simulink model "abe_simulink_model"  (R2022a)
settings: Solver=VariableStepAuto  StartTime=0.0  StopTime=50  RelTol=1e-3
libraries: simulink x1
settings Model: Creator=Abraham  LastModifiedBy=Abraham

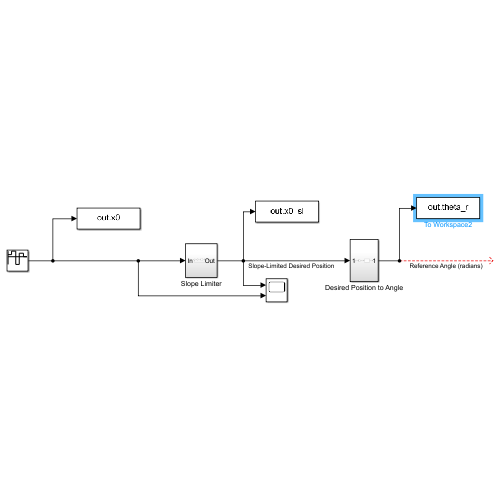
[thumbnail: Simulink's stored preview of the top-level diagram]
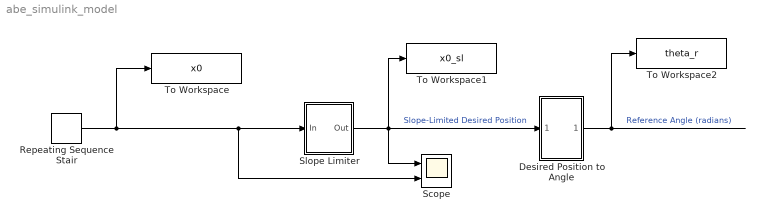
== system abe_simulink_model ==
  Desired Position to Angle : Subsystem
  Repeating Sequence Stair : simulink/Sources/Repeating Sequence Stair  OutValues=[5 15 -20 10 0].'  tsamp=10  OutMin=[]  OutMax=[]  OutDataTypeStr=double  OutputDataTypeScalingMode=double  OutDataType=fixdt(0,8)  ConRadixGroup=Best Precision: Vector-wise  OutScaling=2^-12
  Scope : Scope  NumInputPorts=2
  Slope Limiter : Subsystem
  To Workspace : ToWorkspace  VariableName=x0  SaveFormat=Timeseries  SampleTime=-1
  To Workspace1 : ToWorkspace  VariableName=x0_sl  SaveFormat=Timeseries  SampleTime=-1
  To Workspace2 : ToWorkspace  VariableName=theta_r  SaveFormat=Timeseries  SampleTime=-1
  wires:
  Slope Limiter/1(Out) -> To Workspace1/1, Desired Position to Angle/1(In1), Scope/1  "Slope-Limited Desired Position"
  Repeating Sequence Stair/1 -> To Workspace/1, Scope/2, Slope Limiter/1(In)
  Desired Position to Angle/1(Out1) -> To Workspace2/1  "Reference Angle (radians)"

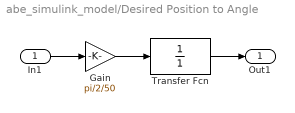
== system abe_simulink_model/Desired Position to Angle ==
  In1 : Inport
  Gain : Gain  Gain=pi/2/50
  Transfer Fcn : TransferFcn  Denominator=[1]
  Out1 : Outport
  wires:
  Gain/1 -> Transfer Fcn/1
  In1/1 -> Gain/1
  Transfer Fcn/1 -> Out1/1

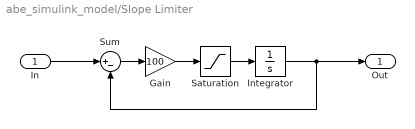
== system abe_simulink_model/Slope Limiter ==
  In : Inport
  Gain : Gain  Gain=100
  Integrator : Integrator
  Saturation : Saturate  UpperLimit=10  LowerLimit=-10
  Sum : Sum  Inputs=|+-
  Out : Outport
  wires:
  Integrator/1 -> Out/1, Sum/2
  Gain/1 -> Saturation/1
  Saturation/1 -> Integrator/1
  Sum/1 -> Gain/1
  In/1 -> Sum/1
